simulink model "Simulink_Model_final"  (R2025a)
settings: Solver=VariableStepAuto  StartTime=0.0  StopTime=5.0  RelTol=1e-3
libraries: simulink x1, simulink_extras x1
settings Model: Creator=shami  LastModifiedBy=shami

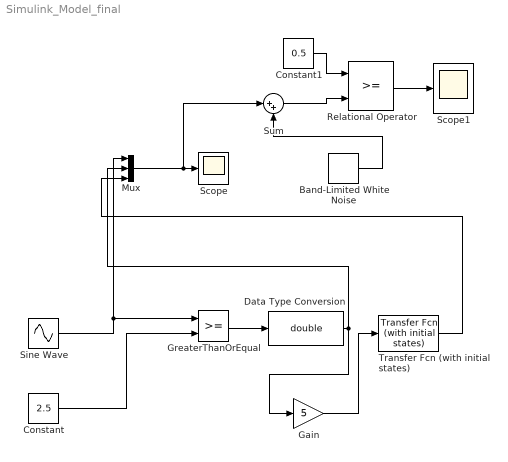
== system Simulink_Model_final ==
  Band-Limited White Noise : simulink/Sources/Band-Limited White Noise  Cov=0.05  Ts=0.01  seed=[12345]
  Constant : Constant  Value=2.5
  Constant1 : Constant  Value=0.5
  Data Type Conversion : DataTypeConversion  OutDataTypeStr=double  SaturateOnIntegerOverflow=off  RndMeth=Floor
  Gain : Gain  Gain=5
  GreaterThanOrEqual : RelationalOperator  OutDataTypeStr=boolean  RndMeth=Simplest  InputSameDT=off
  Mux : Mux  Inputs=3
  Relational Operator : RelationalOperator  OutDataTypeStr=boolean  RndMeth=Simplest  InputSameDT=off
  Scope : Scope
      settings: ActiveDisplayYMinimum=-0.78296865287496686  ActiveDisplayYMaximum=5.3399272032932013
  Scope1 : Scope
      settings: ActiveDisplayYMinimum=0.67393577824220174  ActiveDisplayYMaximum=0.715363837337634
  Sine Wave : Sin  Amplitude=2.5  Bias=2.5  Frequency=2*pi*1000  SampleTime=0
  Sum : Sum  Inputs=|++
  Transfer Fcn (with initial states) : simulink_extras/Additional Linear/Transfer Fcn (with initial states)  N=[1]  D="[0.01  1]"  X0=0
  wires:
  Sine Wave/1 -> Mux/1, GreaterThanOrEqual/1
  Constant/1 -> GreaterThanOrEqual/2
  GreaterThanOrEqual/1 -> Data Type Conversion/1
  Gain/1 -> Transfer Fcn (with initial states)/1
  Data Type Conversion/1 -> Gain/1, Mux/2
  Mux/1 -> Sum/1, Scope/1
  Transfer Fcn (with initial states)/1 -> Mux/3
  Sum/1 -> Relational Operator/2
  Band-Limited White Noise/1 -> Sum/2
  Constant1/1 -> Relational Operator/1
  Relational Operator/1 -> Scope1/1
